simulink model "IARC_Nonlinear_Sensors"  (R2018a)
settings: Solver=ode1  StartTime=0.0  StopTime=20  FixedStep=T  RelTol=1e-3  EnableMultiTasking=on
undefined symbols (not defined in the file): A_1df, A_2df, alpha3, alpha_rp, alpha_x, alpha_z, an1, an1_v, an2, an3, bn1, bn1_v, bn2, bn3, dc_M_x, delta3, Epsilon3, F, g, Gamma1, Gamma2, Gamma3, Gamma4, gamma4_0, gamma_d_x, gamma_rp_0, gamma_x_0, gamma_z_0, Gammax, I, I_add, I_add_time, Jx, Jy, Jyaw, K, k1, k10, k11, k12, k2, k3, k4, k5, k6, k7, k8, k9, Ky, L, Light, LIMIT_CMD_PITCH, LIMIT_CMD_ROLL, LIMIT_CMD_xy, LIMIT_uCMD_HEIGHT, m, m_add, m_add_time, magnitude, MIL ... (+67)
libraries: simulink x131, simulink_extras x5, UAV_Control x4, aerolibwind2 x1
(part 4 of 6)

== system IARC_Nonlinear_Sensors/ARC Controller/Position Control/Z control/Estimate theta = K//m ==
  Phi_d : Inport
  error : Inport  Port=2
  f(f) : Inport  Port=3
  Phi : Inport  Port=4
  adappt : Inport  Port=5
  1 : Scope
  11 : Scope
  Constant4 : Constant  Value=6.7
  Constant6 : Constant  Value=theta3_Max(1,1)
  Constant7 : Constant  Value=theta3_Min(1,1)
  Demux1 : Demux  Outputs=2
  Demux2 : Demux  Outputs=2
  Gain1 : Gain  Gain=K
  "IARC, Physical Model Based Parameter Estimation (69)" : Subsystem  AncestorBlock=|  mask(Physical Model Based Parameter Estimation){mu1=mu1_z, mu2=mu2_z, alpha=alpha_z, nu=nu_z, gamma0=gamma_z_0, Rho_M=Rho_M_z, Rho_L=Rho_L_z, v=v_z, theta_0=theta3_0, theta_max=theta3_Max, theta_min=theta3_Min, Theta_dot_M=theta_dot_M_z, Tau=Tau_z, t0=t0, Norm_ON=on}
      | UAV_Control/IARC, Physical Model Based 
      | Parameter Estimation (69)
      mask prompts: mu1 "forgetting factor, mu1:"; mu2 "RLS parameter, mu2:"; alpha "forgetting factor, alpha:"; nu "normalizing factor, nu:"; gamma0 "Initial adaptation gain:"; Rho_M "Upper bound for the adaptation gain:"; Rho_L "Lower bound for the adaptation gain:"; v "Eigenvector of Gamma_max:"; Theta_dot_M "Theta dot max:"; Tau "Filter time constant:"; t0 "Initialization Delay:"; Norm_ON "Use Normalized formula"
      mask Help:
      | Filtered system dynamics:
      | H_f (s)  is any stable LTI filter transfer function
      | x_f=H_f [x]
      | φ_f=H_f [φ(x)]
      | u_f=H_f [u]
      | 
      | y_p=x ̇_f−u_f
      | y ̂_p=φ_f^T θ ̂
      | Prediction error:
      | ϵ=y_p−y ̂_p
      | 
      | recursive estimation algorithms, the generalized parameter estimation algorithm (PAA) with covariance limiting:
      | 
      | θ ̂  ̇(t)=Γ(t) φ_f (t)ϵ(t)
      | D_Γ=μ_1 (t)Γ(t)−μ_2 (t)Γ(t) φ_f (t) φ_f (t)^T Γ(t)
      | Γ ̇(t)=D_Γ, if λ_M (Γ(t))<ρ_M  or v_M^T D_Γ v_M<0 )
      |          0        else
      | 
      | μ_1  and μ_2  are two non-negative functions
      | ρ_M  is a preset upper bound for the covariance matrix Γ(t)
      | μ_1  represents the forgetting factor (μ_1=0 for not forgetting)
      | μ_2: 1 stands for the standard least squares type estimation algorithm
      |        0 stands for  the gradient type estimation algorithm
      |        range: 0≤μ_2<2
      | Initialization of the covariance matrix: Γ(0)<ρ_M I_p
      | 
      | IARC designs completely separate the parameter estimation law design from the underlying robust control law to give better parameter estimates than possible with DARC designs. In addition, explicit on-line signal excitation level monitoring can be employed to significantly improve the accuracy of  parameter estimates.
      | 
      | Normalized Method:
      | θ ̂  ̇(t)=(Γ(t) φ_f (t)ϵ(t))/(1+νφ_f^T Γφ_f )
      | D_Γ=αΓ(t)−(Γ(t) φ_f (t) φ_f (t)^T Γ(t))/(1+νφ_f^T Γφ_f )
      | Γ ̇(t)=D_Γ, if λ_M (Γ(t))<ρ_M  or v_M^T D_Γ v_M<0
      |           0       else
      mask Display:
      | port_label('input',1,'y','texmode','on')
      | port_label('input',2,'\phi','texmode','on')
      | port_label('input',3,'Adapt','texmode','on')
      | 
      | port_label('output',1,'\theta_{hat}','texmode','on')
  Integral Type Adaptation Law Discontinuous Projection : Subsystem  AncestorBlock=|  mask(IntegralTypeAdaptationLaw){theta=theta3(1,1), theta0=theta3_0(1,1), theta_max=theta3_Max(1,1), theta_min=theta3_Min(1,1), gamma=Gamma3(1,1), t0=3, Adaptation_ON=on}
      | UAV_Control/Integral Type
      | Adaptation Law
      | Discontinuous Projection
      mask prompts: theta "Actual value of theta:"; theta0 "Initial value of theta:"; theta_max "Maximum value of theta:"; theta_min "Minimum value of theta:"; gamma "Adaptation Rate:"; t0 "Initialization Delay:"; Adaptation_ON "Activate adaptation:"
      mask help: Applies an Integral-type adaptation law with discontinuous projection on the parameter theta.
      mask Help:
      | Applies an Integral-type adaptation law with discontinuous projection on the parameter theta.
      | 
      | theta_est_dot=Gamma*Phi*e
      | theta=proj( int(theta_estdot) )
      | 
      | theta_min < theta_est <  theta_max
      | 
      | Parameters:
      | 
      | Gamma: nxn diagonal matrix, adaptaion rate.
      | theta_min: nx1 vector, minimum value of the estimated vector.
      | theta_max: nx1 vector, maximum value of the estimated vector.
      | theta0: nx1 vector, initial value of the estimated vector.
      | theta: nx1 vector, actual value of the estimated vector.
      | Adaptation_On: controls the use of the adaptation law (1: active, 0: inactive)
      | 
      | Inputs:
      | Phi: regressor vector, theta0, nx1.
      | e: state error, scalar.
      | 
      | Outputs:
      | theta_est: estimated value of the parameters vector.
      mask Display:
      | port_label('input',1,'\phi','texmode','on')
      | port_label('input',2,'e','texmode','on')
      | port_label('output',1,'\theta_{hat}','texmode','on')
  Manual Switch : ManualSwitch  CurrentSetting=0
  Manual Switch1 : ManualSwitch
  Math Function1 : Math  Operator=reciprocal  SaturateOnIntegerOverflow=on
  Mux8 : Mux  Inputs=5
  To File : ToFile  Commented=on  Filename=IARC31.mat  MatrixName=IARC31  SaveFormat=Timeseries
  To Workspace2 : ToWorkspace  Commented=on  VariableName=theta_3  SaveFormat=Timeseries  SampleTime=-1
  m : Subsystem
  m (kg) : Scope
  theta1 : Outport
  theta2 : Outport  Port=2
  wires:
  Phi/1 -> "IARC, Physical Model Based Parameter Estimation (69)"/2(Phi)
  Constant6/1 -> Mux8/4
  Integral Type Adaptation Law Discontinuous Projection/1(theta_est) -> 11/1, Mux8/1, Manual Switch/1
  Demux2/1 -> Manual Switch/2, Mux8/2
  m/1(Out1) -> Mux8/3
  Math Function1/1 -> Gain1/1
  error/1 -> Integral Type Adaptation Law Discontinuous Projection/2(error)
  Manual Switch/1 -> 1/1, theta1/1, To Workspace2/1
  Constant7/1 -> Mux8/5
  Gain1/1 -> To File/1, m (kg)/1
  Mux8/1 -> Math Function1/1
  Phi_d/1 -> Integral Type Adaptation Law Discontinuous Projection/1(Phi)
  f(f)/1 -> "IARC, Physical Model Based Parameter Estimation (69)"/1(y)
  adappt/1 -> "IARC, Physical Model Based Parameter Estimation (69)"/3(Adapt1)
  Manual Switch1/1 -> theta2/1
  "IARC, Physical Model Based Parameter Estimation (69)"/1(Theta_hat) -> Demux2/1
  Demux1/2 -> Manual Switch1/1
  Demux2/2 -> Manual Switch1/2

== system IARC_Nonlinear_Sensors/ARC Controller/Position Control/Z control/Phi ==
  "  " : Gain  Gain=1/K
  Constant : Constant
  Mux1 : Mux  Inputs=2
  Mux2 : Mux  Inputs=2
  Product1 : Product
  cos : Trigonometry  Operator=cos
  cos(phi).cos(theta) : Fcn  Expr=u(1)*u(2)
  rotor TF : TransferFcn  Numerator=1  Denominator=[Tm 1]
  Out1 : Outport
  wires:
  Mux2/1 -> cos/1
  [phi] -> Mux2/1
  cos(phi).cos(theta)/1 -> Product1/1
  [theta] -> Mux2/2
  rotor TF/1 -> Product1/2
  Mux1/1 -> Out1/1
  Product1/1 -> Mux1/1
  Constant/1 -> Mux1/2
  [Fz_des] -> "  "/1
  cos/1 -> cos(phi).cos(theta)/1
  "  "/1 -> rotor TF/1

== system IARC_Nonlinear_Sensors/ARC Controller/Position Control/Z control/Phi1 ==
  "  " : Gain  Gain=1/K
  Fcn33 : Fcn  Expr=u(4)*u(5)
  Mux : Mux  Inputs=2
  Mux2 : Mux  Inputs=3
  Product1 : Product
  rotor2 : TransferFcn  Numerator=1  Denominator=[Tm 1]
  sincos : Trigonometry  Operator=sincos
  Out1 : Outport
  wires:
  Product1/1 -> Out1/1
  rotor2/1 -> Product1/2
  [theta] -> Mux2/2
  Fcn33/1 -> Product1/1
  sincos/1 -> Mux/1
  sincos/2 -> Mux/2
  [psi] -> Mux2/3
  Mux/1 -> Fcn33/1
  [phi] -> Mux2/1
  Mux2/1 -> sincos/1
  [Fz_des] -> "  "/1
  "  "/1 -> rotor2/1

== system IARC_Nonlinear_Sensors/ARC Controller/Position Control/Z control/Phi3 ==
  "  " : Gain  Gain=1/K
  Constant : Constant
  Mux1 : Mux  Inputs=2
  Mux2 : Mux  Inputs=2
  Product1 : Product
  cos : Trigonometry  Operator=cos
  cos(phi).cos(theta) : Fcn  Expr=u(1)*u(2)
  rotor TF : TransferFcn  Numerator=1  Denominator=[Tm 1]
  Out1 : Outport
  wires:
  cos/1 -> cos(phi).cos(theta)/1
  [Fz_des] -> "  "/1
  Constant/1 -> Mux1/2
  Product1/1 -> Mux1/1
  Mux1/1 -> Out1/1
  rotor TF/1 -> Product1/2
  [theta] -> Mux2/2
  cos(phi).cos(theta)/1 -> Product1/1
  [phi] -> Mux2/1
  Mux2/1 -> cos/1
  "  "/1 -> rotor TF/1

== system IARC_Nonlinear_Sensors/ARC Controller/Position Control/Z control/e10 ==
  Add : Sum
  Discrete Derivative2 : simulink/Discrete/Discrete Derivative  gainval=1.0  ICPrevScaledInput=0.0  OutMin=[]  OutMax=[]  OutDataType=fixdt(1, 16)  OutScaling=2^-10  DoSatur=off
  Sum1 : Sum  Inputs=-+|
  Sum3 : Sum  Inputs=|+-
  k9 : Gain  Gain=k9
  e10 : Outport
  wires:
  k9/1 -> Add/1
  Discrete Derivative2/1 -> Sum1/1
  [z_dot] -> Sum1/2
  Add/1 -> e10/1
  Sum3/1 -> k9/1  "ex"
  Sum1/1 -> Add/2  "ev"
  [z] -> Sum3/1
  [z_des] -> Discrete Derivative2/1, Sum3/2

== system IARC_Nonlinear_Sensors/ARC Controller/Position Control/Z control/f(x) ==
  Add : Sum
  Constant : Constant  Value=g
  Discrete Derivative1 : simulink/Discrete/Discrete Derivative  gainval=1.0  ICPrevScaledInput=0.0  OutMin=[]  OutMax=[]  OutDataType=fixdt(1, 16)  OutScaling=2^-10  DoSatur=off
  Out1 : Outport
  wires:
  Add/1 -> Out1/1
  [z_dot] -> Discrete Derivative1/1
  Discrete Derivative1/1 -> Add/1
  Constant/1 -> Add/2

== system IARC_Nonlinear_Sensors/Sensors and Filters/Data processing/Estimate Attitude/2nd Order Filter3 ==
  u : Inport
  "  1" : Constant  Value=OMEGA_FILTER_OUTER
  "  2" : Constant  Value=2
  "  zea" : Constant
  Integrator : Integrator
  Integrator1 : Integrator
  Product : Product
  Product1 : Product
  Product2 : Product  Inputs=3
  Sum : Sum  Inputs=|+-
  Sum1 : Sum  Inputs=|+-
  y : Outport
  yd : Outport  Port=2
  wires:
  Product2/1 -> Sum1/2
  "  zea"/1 -> Product2/3
  "  2"/1 -> Product2/2
  Product1/1 -> Integrator1/1, yd/1
  Integrator1/1 -> y/1, Sum/2
  u/1 -> Sum/1
  Sum1/1 -> Product/2
  "  1"/1 -> Product/1, Product1/1
  Product/1 -> Integrator/1
  Integrator/1 -> Product1/2, Product2/1
  Sum/1 -> Sum1/1

== system IARC_Nonlinear_Sensors/Sensors and Filters/Data processing/Estimate Attitude/Calculate Roll and Pitch (From Acceleration Data) ==
  accel (m/s^2) [3] : Inport
  Gain{1..2,6..7} (4 alike) : Gain  Commented=on  Gain=180/pi
  Gain3 : Gain
  calc_roll_pitch : MATLAB Function  TreatAsAtomicUnit=on
  calc_roll_pitch_asin : MATLAB Function  Commented=on  TreatAsAtomicUnit=on
  pitch_acc : Scope  Commented=on
  pitch_acc_asin : Scope  Commented=on
  roll_acc : Scope  Commented=on
  roll_acc_asin : Scope  Commented=on
  roll_acc (rad) : Outport
  pitch_acc (rad) : Outport  Port=2
  wires:
  accel (m/s^2) [3]/1 -> calc_roll_pitch_asin/1(acc_body), calc_roll_pitch/1(acc_body)
  calc_roll_pitch/1(roll_acc) -> roll_acc (rad)/1, Gain2/1
  calc_roll_pitch/2(pitch_acc) -> Gain3/1, Gain1/1
  Gain2/1 -> roll_acc/1
  Gain1/1 -> pitch_acc/1
  calc_roll_pitch_asin/1(roll_acc) -> Gain6/1
  Gain6/1 -> roll_acc_asin/1
  calc_roll_pitch_asin/2(pitch_acc) -> Gain7/1
  Gain7/1 -> pitch_acc_asin/1
  Gain3/1 -> pitch_acc (rad)/1

== system IARC_Nonlinear_Sensors/Sensors and Filters/Data processing/Estimate Attitude/Notch Filter1 ==
  u : Inport
  Discrete Transfer Fcn : DiscreteTransferFcn  Numerator=an1  Denominator=bn1  SampleTime=1/500
  Discrete Transfer Fcn1 : DiscreteTransferFcn  Numerator=an2  Denominator=bn2  SampleTime=1/500
  Discrete Transfer Fcn2 : DiscreteTransferFcn  Numerator=an3  Denominator=bn3  SampleTime=1/500
  First-Order Hold : simulink/Discrete/First-Order Hold  DisableCoverage=on  Ts=1/500
      settings: SourceProductName=Simulink  SourceProductBaseCode=SL
  Mux : Mux  Commented=on
  Mux1 : Mux  Commented=on  Inputs=2
  Scope : Scope  Commented=on
  Scope1 : Scope  Commented=on
  Transfer Fcn : TransferFcn  Numerator=[60]  Denominator=[1 60]
  y : Outport
  q : Outport  Port=2
  wires:
  u/1 -> Mux1/1, Transfer Fcn/1
  Transfer Fcn/1 -> Mux1/2, First-Order Hold/1, y/1
  Discrete Transfer Fcn1/1 -> Mux/3, Discrete Transfer Fcn2/1
  First-Order Hold/1 -> Discrete Transfer Fcn/1, Mux/1
  Mux/1 -> Scope/1
  Discrete Transfer Fcn/1 -> Mux/2, Discrete Transfer Fcn1/1
  Mux1/1 -> Scope1/1
  Discrete Transfer Fcn2/1 -> q/1, Mux/4

== system IARC_Nonlinear_Sensors/Sensors and Filters/Data processing/Estimate Attitude/Notch Filter2 ==
  u : Inport
  Discrete Transfer Fcn : DiscreteTransferFcn  Numerator=an1  Denominator=bn1  SampleTime=1/500
  Discrete Transfer Fcn1 : DiscreteTransferFcn  Numerator=an2  Denominator=bn2  SampleTime=1/500
  Discrete Transfer Fcn2 : DiscreteTransferFcn  Numerator=an3  Denominator=bn3  SampleTime=1/500
  First-Order Hold : simulink/Discrete/First-Order Hold  DisableCoverage=on  Ts=1/500
      settings: SourceProductName=Simulink  SourceProductBaseCode=SL
  Mux : Mux  Commented=on
  Mux1 : Mux  Commented=on  Inputs=2
  Scope : Scope  Commented=on
  Scope1 : Scope  Commented=on
  To File : ToFile  Commented=on  Filename=P_gyro_Noisy.mat  MatrixName=P_gyro_Noisy  SaveFormat=Timeseries
  Transfer Fcn : TransferFcn  Numerator=[60]  Denominator=[1 60]
  y : Outport
  p : Outport  Port=2
  wires:
  Mux1/1 -> Scope1/1
  Discrete Transfer Fcn/1 -> Discrete Transfer Fcn1/1, Mux/2
  Discrete Transfer Fcn2/1 -> p/1, Mux/4
  Mux/1 -> Scope/1
  First-Order Hold/1 -> Mux/1, Discrete Transfer Fcn/1
  Discrete Transfer Fcn1/1 -> Discrete Transfer Fcn2/1, Mux/3
  Transfer Fcn/1 -> y/1, First-Order Hold/1, Mux1/2
  u/1 -> To File/1, Transfer Fcn/1, Mux1/1

== system IARC_Nonlinear_Sensors/Sensors and Filters/Data processing/Estimate Attitude/Notch Filter3 ==
  u : Inport
  Discrete Transfer Fcn : DiscreteTransferFcn  Numerator=an1  Denominator=bn1  SampleTime=1/500
  Discrete Transfer Fcn1 : DiscreteTransferFcn  Numerator=an2  Denominator=bn2  SampleTime=1/500
  Discrete Transfer Fcn2 : DiscreteTransferFcn  Numerator=an3  Denominator=bn3  SampleTime=1/500
  First-Order Hold : simulink/Discrete/First-Order Hold  DisableCoverage=on  Ts=1/500
      settings: SourceProductName=Simulink  SourceProductBaseCode=SL
  Mux : Mux  Commented=on
  Mux1 : Mux  Commented=on  Inputs=2
  Scope : Scope  Commented=on
  Scope1 : Scope  Commented=on
  Transfer Fcn : TransferFcn  Numerator=[60]  Denominator=[1 60]
  y : Outport
  r : Outport  Port=2
  wires:
  u/1 -> Mux1/1, Transfer Fcn/1
  Transfer Fcn/1 -> Mux1/2, First-Order Hold/1, y/1
  Discrete Transfer Fcn1/1 -> Mux/3, Discrete Transfer Fcn2/1
  First-Order Hold/1 -> Discrete Transfer Fcn/1, Mux/1
  Mux/1 -> Scope/1
  Discrete Transfer Fcn2/1 -> r/1, Mux/4
  Discrete Transfer Fcn/1 -> Mux/2, Discrete Transfer Fcn1/1
  Mux1/1 -> Scope1/1

== system IARC_Nonlinear_Sensors/Sensors and Filters/Data processing/Estimate Position/2nd Order Filter ==
  u : Inport
  "  2" : Constant  Value=2
  "  wn" : Constant  Value=OMEGA_FILTER_OUTER
  "  zea" : Constant
  Integrator : Integrator
  Integrator1 : Integrator
  Product : Product
  Product1 : Product
  Product2 : Product  Inputs=3
  Sum : Sum  Inputs=|+-
  Sum1 : Sum  Inputs=|+-
  y : Outport
  yd : Outport  Port=2
  wires:
  Sum/1 -> Sum1/1
  Integrator/1 -> Product2/1, Product1/2
  Product/1 -> Integrator/1
  "  wn"/1 -> Product1/1, Product/1
  Sum1/1 -> Product/2
  u/1 -> Sum/1
  Integrator1/1 -> Sum/2, y/1
  Product1/1 -> yd/1, Integrator1/1
  "  2"/1 -> Product2/2
  "  zea"/1 -> Product2/3
  Product2/1 -> Sum1/2

== system IARC_Nonlinear_Sensors/Sensors and Filters/Data processing/Estimate Position/2nd Order Filter1 ==
  u : Inport
  "  2" : Constant  Value=2
  "  wn" : Constant  Value=OMEGA_FILTER_OUTER
  "  zea" : Constant
  Integrator : Integrator
  Integrator1 : Integrator
  Product : Product
  Product1 : Product
  Product2 : Product  Inputs=3
  Sum : Sum  Inputs=|+-
  Sum1 : Sum  Inputs=|+-
  y : Outport
  yd : Outport  Port=2
  wires:
  Product2/1 -> Sum1/2
  "  zea"/1 -> Product2/3
  "  2"/1 -> Product2/2
  Product1/1 -> Integrator1/1, yd/1
  Integrator1/1 -> y/1, Sum/2
  u/1 -> Sum/1
  Sum1/1 -> Product/2
  "  wn"/1 -> Product/1, Product1/1
  Product/1 -> Integrator/1
  Integrator/1 -> Product1/2, Product2/1
  Sum/1 -> Sum1/1

== system IARC_Nonlinear_Sensors/Sensors and Filters/Data processing/Estimate Position/2nd Order Filter2 ==
  u : Inport
  "  2" : Constant  Value=2
  "  wn" : Constant  Value=OMEGA_FILTER_OUTER
  "  zea" : Constant
  Integrator : Integrator
  Integrator1 : Integrator
  Product : Product
  Product1 : Product
  Product2 : Product  Inputs=3
  Sum : Sum  Inputs=|+-
  Sum1 : Sum  Inputs=|+-
  y : Outport
  yd : Outport  Port=2
  wires:
  Sum/1 -> Sum1/1
  Integrator/1 -> Product2/1, Product1/2
  Product/1 -> Integrator/1
  "  wn"/1 -> Product1/1, Product/1
  Sum1/1 -> Product/2
  u/1 -> Sum/1
  Integrator1/1 -> Sum/2, y/1
  Product1/1 -> yd/1, Integrator1/1
  "  2"/1 -> Product2/2
  "  zea"/1 -> Product2/3
  Product2/1 -> Sum1/2

== system IARC_Nonlinear_Sensors/Sensors and Filters/Data processing/Estimate Position/2nd Order Filter4 ==
  u : Inport
  "  1" : Constant  Value=OMEGA_FILTER_OUTER
  "  2" : Constant  Value=2
  "  zea" : Constant
  Integrator : Integrator
  Integrator1 : Integrator
  Product : Product
  Product1 : Product
  Product2 : Product  Inputs=3
  Sum : Sum  Inputs=|+-
  Sum1 : Sum  Inputs=|+-
  y : Outport
  yd : Outport  Port=2
  wires:
  Product2/1 -> Sum1/2
  "  zea"/1 -> Product2/3
  "  2"/1 -> Product2/2
  Product1/1 -> Integrator1/1, yd/1
  Integrator1/1 -> y/1, Sum/2
  u/1 -> Sum/1
  Sum1/1 -> Product/2
  "  1"/1 -> Product/1, Product1/1
  Product/1 -> Integrator/1
  Integrator/1 -> Product1/2, Product2/1
  Sum/1 -> Sum1/1

== system IARC_Nonlinear_Sensors/Sensors and Filters/Data processing/Estimate Position/2nd Order Filter5 ==
  u : Inport
  "  2" : Constant  Value=2
  "  wn" : Constant  Value=OMEGA_FILTER_OUTER
  "  zea" : Constant
  Integrator : Integrator
  Integrator1 : Integrator
  Product : Product
  Product1 : Product
  Product2 : Product  Inputs=3
  Sum : Sum  Inputs=|+-
  Sum1 : Sum  Inputs=|+-
  y : Outport
  yd : Outport  Port=2
  wires:
  Product2/1 -> Sum1/2
  "  zea"/1 -> Product2/3
  "  2"/1 -> Product2/2
  Product1/1 -> Integrator1/1, yd/1
  Integrator1/1 -> y/1, Sum/2
  u/1 -> Sum/1
  Sum1/1 -> Product/2
  "  wn"/1 -> Product/1, Product1/1
  Product/1 -> Integrator/1
  Integrator/1 -> Product1/2, Product2/1
  Sum/1 -> Sum1/1

== system IARC_Nonlinear_Sensors/Sensors and Filters/Data processing/Estimate Position/Notch Filter1 ==
  u : Inport
  Discrete Transfer Fcn : DiscreteTransferFcn  Numerator=an1_v  Denominator=bn1_v  SampleTime=1/500
  First-Order Hold : simulink/Discrete/First-Order Hold  DisableCoverage=on  Ts=1/500
      settings: SourceProductName=Simulink  SourceProductBaseCode=SL
  Mux : Mux  Commented=on  Inputs=3
  Scope : Scope  Commented=on
  Transfer Fcn : TransferFcn  Numerator=[60]  Denominator=[1 60]
  y : Outport
  wires:
  u/1 -> Transfer Fcn/1, Mux/1
  First-Order Hold/1 -> Discrete Transfer Fcn/1, Mux/2
  Mux/1 -> Scope/1
  Discrete Transfer Fcn/1 -> y/1, Mux/3
  Transfer Fcn/1 -> First-Order Hold/1

== system IARC_Nonlinear_Sensors/Sensors and Filters/Data processing/Estimate Position/Notch Filter2 ==
  u : Inport
  Discrete Transfer Fcn : DiscreteTransferFcn  Numerator=an1_v  Denominator=bn1_v  SampleTime=1/500
  First-Order Hold : simulink/Discrete/First-Order Hold  DisableCoverage=on  Ts=1/500
      settings: SourceProductName=Simulink  SourceProductBaseCode=SL
  Mux : Mux  Commented=on  Inputs=3
  Scope : Scope  Commented=on
  Transfer Fcn : TransferFcn  Numerator=[60]  Denominator=[1 60]
  y : Outport
  wires:
  Discrete Transfer Fcn/1 -> y/1, Mux/3
  Mux/1 -> Scope/1
  First-Order Hold/1 -> Mux/2, Discrete Transfer Fcn/1
  u/1 -> Mux/1, Transfer Fcn/1
  Transfer Fcn/1 -> First-Order Hold/1

== system IARC_Nonlinear_Sensors/Sensors and Filters/Data processing/Estimate Position/Signal Conditioning - Sonar ==
  note: Correct for Roll and Pitch
  note: "Smooth" out the Sonar data
  note: Resample the 10Hz Sonar Data
  sonar (m) : Inport
  roll (rad) : Inport  Port=2
  pitch (rad) : Inport  Port=3
  FOH1 : Subsystem  mask{Ts=0.1}
      mask prompts: Ts "Sample Time"
  "Height Estimate Bias (Estimate Reference at Centre of QBall 2) " : Bias
  Product : Product  Inputs=3  RndMeth=Zero
  Rate Transition : RateTransition
  Sampler : Subsystem  mask{Ts=0.1}
      mask prompts: Ts "Sample Time"
  Trigonometric Function : Trigonometry  Operator=cos
  Trigonometric Function2 : Trigonometry  Operator=cos
  calib sonar (m) : Outport
  wires:
  Sampler/1(Out1) -> Rate Transition/1
  Rate Transition/1 -> FOH1/1(Input)
  sonar (m)/1 -> Sampler/1(In1)
  FOH1/1(Output) -> Product/1
  Trigonometric Function2/1 -> Product/2
  roll (rad)/1 -> Trigonometric Function2/1
  pitch (rad)/1 -> Trigonometric Function/1
  Trigonometric Function/1 -> Product/3
  Product/1 -> "Height Estimate Bias (Estimate Reference at Centre of QBall 2) "/1
  "Height Estimate Bias (Estimate Reference at Centre of QBall 2) "/1 -> calib sonar (m)/1

== system IARC_Nonlinear_Sensors/ARC Controller/Attitutde Control/Subsystem/f/d(T)//d(phi) ==
  R1,R2,R3 : Inport  PortDimensions=3
  Fcn{1,11..13,22,32} (6 alike) : Fcn  Expr=0
  Fcn2 : Fcn  Expr=u(4)
  Fcn3 : Fcn  Expr=-u(1)*u(5)
  Fcn31 : Fcn  Expr=u(1)*u(2)
  Mux : Mux  Inputs=2
  Subsystem : Subsystem
  sincos : Trigonometry  Operator=sincos
  T : Outport  PortDimensions=[3,3]
  wires:
  Fcn3/1 -> Subsystem/9(In9)
  Fcn2/1 -> Subsystem/8(In8)
  Fcn1/1 -> Subsystem/6(In6)
  Fcn22/1 -> Subsystem/5(In5)
  Fcn31/1 -> Subsystem/7(In7)
  Fcn32/1 -> Subsystem/4(In4)
  Fcn13/1 -> Subsystem/3(In3)
  Fcn12/1 -> Subsystem/2(In2)
  Fcn11/1 -> Subsystem/1(In1)
  Mux/1 -> Fcn1/1, Fcn31/1, Fcn3/1, Fcn2/1, Fcn32/1, Fcn12/1, Fcn11/1, Fcn13/1, Fcn22/1
  sincos/2 -> Mux/2
  sincos/1 -> Mux/1
  Subsystem/1(Out1) -> T/1
  R1,R2,R3/1 -> sincos/1

== system IARC_Nonlinear_Sensors/ARC Controller/Attitutde Control/Subsystem/f/d(T)//d(theta) ==
  R1,R2,R3 : Inport  PortDimensions=3
  Fcn{1..2,12,22,32} (5 alike) : Fcn  Expr=0
  Fcn11 : Fcn  Expr=-u(2)
  Fcn13 : Fcn  Expr=u(5)
  Fcn3 : Fcn  Expr=-u(4)*u(2)
  Fcn31 : Fcn  Expr=-u(4)*u(5)
  Mux : Mux  Inputs=2
  Subsystem : Subsystem
  sincos : Trigonometry  Operator=sincos
  T : Outport  PortDimensions=[3,3]
  wires:
  R1,R2,R3/1 -> sincos/1
  Subsystem/1(Out1) -> T/1
  sincos/1 -> Mux/1
  sincos/2 -> Mux/2
  Mux/1 -> Fcn22/1, Fcn13/1, Fcn11/1, Fcn12/1, Fcn32/1, Fcn2/1, Fcn3/1, Fcn31/1, Fcn1/1
  Fcn11/1 -> Subsystem/1(In1)
  Fcn12/1 -> Subsystem/2(In2)
  Fcn13/1 -> Subsystem/3(In3)
  Fcn32/1 -> Subsystem/4(In4)
  Fcn31/1 -> Subsystem/7(In7)
  Fcn22/1 -> Subsystem/5(In5)
  Fcn1/1 -> Subsystem/6(In6)
  Fcn2/1 -> Subsystem/8(In8)
  Fcn3/1 -> Subsystem/9(In9)

== system IARC_Nonlinear_Sensors/ARC Controller/Attitutde Control/Yaw control/Phi3/alpha 42 dot ==
  Add : Sum  Inputs=-+
  Discrete Derivative1 : simulink/Discrete/Discrete Derivative  gainval=1.0  ICPrevScaledInput=0.0  OutMin=[]  OutMax=[]  OutDataType=fixdt(1, 16)  OutScaling=2^-10  DoSatur=off
  Discrete Derivative2 : simulink/Discrete/Discrete Derivative  gainval=1.0  ICPrevScaledInput=0.0  OutMin=[]  OutMax=[]  OutDataType=fixdt(1, 16)  OutScaling=2^-10  DoSatur=off
  Sum3 : Sum  Inputs=|+-
  Transfer Fcn3 : TransferFcn  Denominator=A_2df
  k11 : Gain  Gain=k11
  alpha_42_dot : Outport
  wires:
  [psi_des] -> Sum3/2, Discrete Derivative2/1
  [psi] -> Sum3/1
  Sum3/1 -> k11/1  "ex"
  Add/1 -> alpha_42_dot/1
  Discrete Derivative2/1 -> Discrete Derivative1/1
  k11/1 -> Add/1
  Transfer Fcn3/1 -> Add/2
  Discrete Derivative1/1 -> Transfer Fcn3/1

== system IARC_Nonlinear_Sensors/ARC Controller/Attitutde Control/Yaw control/Subsystem/  ==
  1 : Scope  Commented=on
  Constant4 : Constant  Value=Jyaw
  Divide : Product  Inputs=*/
  J_add : Step  Time=I_add_time  After=I_add(3,3)  SampleTime=0
  Selector : Selector  InputPortWidth=3  IndexOptions=Index vector (dialog)  Indices=3  OutputSizes=1
  Sum : Sum  Inputs=|++
  Sum1 : Sum  Inputs=++|
  T_add : Step  Time=T_add_time  After=T_add(1,3)  SampleTime=0
  Out1 : Outport
  wires:
  T_add/1 -> Sum1/2
  [Md] -> Selector/1
  Divide/1 -> 1/1, Out1/1
  Sum/1 -> Divide/2
  Constant4/1 -> Sum/1
  J_add/1 -> Sum/2
  Sum1/1 -> Divide/1
  Selector/1 -> Sum1/1

== system IARC_Nonlinear_Sensors/ARC Controller/Attitutde Control/Yaw control/Subsystem/IARC, Physical Model Based Parameter Estimation (69)_Yaw ==
  f(x) : Inport
  Phi : Inport  Port=2
  Adapt : Inport  Port=3
  Adapt1 : InportShadow  Port=3
  Constant2 : Constant  Value=Norm_ON
  Discontinuous_Proj_(49) : Subsystem
  Display : Display  Commented=on
  Divide : Product  Inputs=*/
  Epsilon : Subsystem
  Filter : Subsystem
  Gamma : Subsystem
  Switch1 : Switch  Threshold=0.5
  Theta_hat_dot : Product  Inputs=3  Multiplication=Matrix(*)
  den : Scope  Commented=on
  "epsilon  " : Scope  Commented=on
  gamma : Scope  Commented=on
  theta dot : Scope  Commented=on
  theta hat : Scope  Commented=on
  Theta_hat : Outport
  wires:
  Epsilon/1(Epsilon) -> Theta_hat_dot/3, "epsilon  "/1  "predicted output error"
  Discontinuous_Proj_(49)/1(Theta) -> theta hat/1, Theta_hat/1, Epsilon/3(Theta_hat)
  Filter/1(f(x)_f) -> Epsilon/1(f(x)_f_dot)
  Phi/1 -> Filter/2("Phi ")
  f(x)/1 -> Filter/1(f(x))
  Theta_hat_dot/1 -> Discontinuous_Proj_(49)/1(Theta_dot), theta dot/1
  Constant2/1 -> Switch1/2
  Gamma/1(" gamma") -> Display/1, gamma/1, Switch1/3, Divide/1
  Switch1/1 -> Theta_hat_dot/1
  Divide/1 -> Switch1/1
  Gamma/2(" 1+nu.Phi.G.Phi") -> den/1, Divide/2
  Filter/2(Phi_f) -> Epsilon/2(Phi_f), Gamma/1(Phi_f), Theta_hat_dot/2
  Adapt/1 -> Gamma/2(Adapt)
  Adapt1/1 -> Discontinuous_Proj_(49)/2(Adapt)

== system IARC_Nonlinear_Sensors/ARC Controller/Attitutde Control/Yaw control/Subsystem/Integral Type Adaptation Law Discontinuous Projection1 ==
  Phi : Inport
  error : Inport  Port=2
  Constant : Constant  Value=gamma
  Constant2 : Constant  Value=Adaptation_ON
  Discontinuous Projection : Integrator  InitialCondition=theta0  LimitOutput=on  UpperSaturationLimit=theta_max  LowerSaturationLimit=theta_min
  InitializationDelay : UAV_Control/InitializationDelay  t0=t0
      settings: SourceProductName=UAV_Control
  Product1 : Product  Inputs=3  Multiplication=Matrix(*)
  Switch1 : Switch  Criteria=u2 ~= 0
  real : Constant  Value=theta
  theta_est : Outport
  wires:
  Constant/1 -> Product1/1
  error/1 -> Product1/3
  real/1 -> Switch1/3
  Constant2/1 -> Switch1/2
  InitializationDelay/1 -> Discontinuous Projection/1
  Product1/1 -> InitializationDelay/1
  Phi/1 -> Product1/2
  Discontinuous Projection/1 -> Switch1/1
  Switch1/1 -> theta_est/1

== system IARC_Nonlinear_Sensors/ARC Controller/Attitutde Control/Yaw control/Subsystem/J ==
  Constant4 : Constant  Value=Jyaw
  Gain : Gain  Gain=Ky
  Math Function : Math  Operator=reciprocal  SaturateOnIntegerOverflow=on
  Step : Step  Time=I_add_time  After=I_add(3,3)  SampleTime=0
  Sum : Sum  Inputs=|++
  Out1 : Outport
  wires:
  Constant4/1 -> Sum/1
  Step/1 -> Sum/2
  Math Function/1 -> Gain/1
  Gain/1 -> Out1/1
  Sum/1 -> Math Function/1

== system IARC_Nonlinear_Sensors/ARC Controller/Attitutde Control/Yaw control/Subsystem/Subsystem1 ==
  u : Inport
  6 : Scope
  Constant4 : Constant  Value=Jy
  Divide : Product  Inputs=**
  J_add : Step  Time=I_add_time  After=I_add(1,1)  SampleTime=0
  Sum : Sum  Inputs=|++
  y : Outport
  wires:
  u/1 -> Divide/1
  J_add/1 -> Sum/2
  Divide/1 -> y/1
  Sum/1 -> Divide/2, 6/1
  Constant4/1 -> Sum/1

== system IARC_Nonlinear_Sensors/ARC Controller/Attitutde Control/Yaw control/f(x)/T1 .. ==
  "  " : Trigonometry  Operator=cos
  "    " : Trigonometry
  Constant : Constant  Value=Jx
  Gain1 : Gain  Gain=-1
  Product1 : Product  Inputs=*/*/
  Out1 : Outport
  wires:
  Product1/1 -> Gain1/1
  Gain1/1 -> Out1/1
  [T1] -> Product1/3
  Constant/1 -> Product1/4
  [phi] -> "  "/1
  [theta] -> "    "/1
  "  "/1 -> Product1/2
  "    "/1 -> Product1/1

== system IARC_Nonlinear_Sensors/ARC Controller/Attitutde Control/Yaw control/f(x)/f ==
  " " : Trigonometry  Operator=sincos
  "  " : Trigonometry
  "      " : Trigonometry  Operator=cos
  Add : Sum  Inputs=++-
  Add1 : Sum  Inputs=+-
  Constant1 : Constant  Value=(Jy-Jyaw)/Jx
  Discrete Derivative1 : simulink/Discrete/Discrete Derivative  gainval=1.0  ICPrevScaledInput=0.0  OutMin=[]  OutMax=[]  OutDataType=fixdt(1, 16)  OutScaling=2^-10  DoSatur=off
  Discrete Derivative2 : simulink/Discrete/Discrete Derivative  gainval=1.0  ICPrevScaledInput=0.0  OutMin=[]  OutMax=[]  OutDataType=fixdt(1, 16)  OutScaling=2^-10  DoSatur=off
  Discrete Derivative3 : simulink/Discrete/Discrete Derivative  gainval=1.0  ICPrevScaledInput=0.0  OutMin=[]  OutMax=[]  OutDataType=fixdt(1, 16)  OutScaling=2^-10  DoSatur=off
  Ground : Ground
  Product1 : Product
  Product2 : Product  Inputs=**/
  Product4 : Product  Inputs=***/
  Selector1 : Selector  InputPortWidth=3  IndexOptions=Index vector (dialog)  Indices=[2 3]  OutputSizes=1
  q.r : Product  Inputs=*
  Out1 : Outport
  wires:
  [phi] -> "      "/1
  "      "/1 -> Product4/4
  Product4/1 -> Add/2
  q.r/1 -> Product4/2
  Selector1/1 -> q.r/1
  [pqr_est] -> Selector1/1
  Constant1/1 -> Product4/1
  Discrete Derivative1/1 -> Product2/1
  " "/2 -> Product2/3
  Add1/1 -> Product2/2
  Product1/1 -> Add1/2
  " "/1 -> Product1/2
  Discrete Derivative2/1 -> Product1/1
  Discrete Derivative3/1 -> Add1/1
  [phi] -> " "/1, Discrete Derivative1/1
  Add/1 -> Out1/1
  Product2/1 -> Add/1
  [theta] -> "  "/1
  "  "/1 -> Product4/3
  [psi] -> Discrete Derivative2/1
  [theta] -> Discrete Derivative3/1
  Ground/1 -> Add/3

== system IARC_Nonlinear_Sensors/ARC Controller/Attitutde Control/Yaw control/phi/Notch Filter2 ==
  u : Inport
  Discrete Transfer Fcn : DiscreteTransferFcn  Numerator=an1  Denominator=bn1  SampleTime=1/500
  Discrete Transfer Fcn1 : DiscreteTransferFcn  Numerator=an2  Denominator=bn2  SampleTime=1/500
  Discrete Transfer Fcn2 : DiscreteTransferFcn  Numerator=an3  Denominator=bn3  SampleTime=1/500
  First-Order Hold : simulink/Discrete/First-Order Hold  DisableCoverage=on  Ts=1/500
      settings: SourceProductName=Simulink  SourceProductBaseCode=SL
  Mux : Mux
  Mux1 : Mux  Inputs=2
  Scope : Scope
  Scope1 : Scope
  Transfer Fcn : TransferFcn  Numerator=[60]  Denominator=[1 60]
  p : Outport
  wires:
  Mux1/1 -> Scope1/1
  Discrete Transfer Fcn/1 -> Discrete Transfer Fcn1/1, Mux/2
  Discrete Transfer Fcn2/1 -> p/1, Mux/4
  Mux/1 -> Scope/1
  First-Order Hold/1 -> Mux/1, Discrete Transfer Fcn/1
  Discrete Transfer Fcn1/1 -> Discrete Transfer Fcn2/1, Mux/3
  Transfer Fcn/1 -> First-Order Hold/1, Mux1/2
  u/1 -> Transfer Fcn/1, Mux1/1

== system IARC_Nonlinear_Sensors/ARC Controller/Attitutde Control/pitch control/Adaptation Law_X/  ==
  1 : Scope
  Constant4 : Constant  Value=Jy
  Divide : Product  Inputs=*/
  J_add : Step  Time=I_add_time  After=I_add(1,1)  SampleTime=0
  Selector : Selector  InputPortWidth=3  IndexOptions=Index vector (dialog)  Indices=2  OutputSizes=1
  Sum : Sum  Inputs=|++
  Sum1 : Sum  Inputs=++|
  T_add : Step  Time=T_add_time  After=T_add(1,2)  SampleTime=0
  Out1 : Outport
  wires:
  T_add/1 -> Sum1/2
  [Md] -> Selector/1
  Divide/1 -> 1/1, Out1/1
  Sum/1 -> Divide/2
  Constant4/1 -> Sum/1
  J_add/1 -> Sum/2
  Sum1/1 -> Divide/1
  Selector/1 -> Sum1/1

== system IARC_Nonlinear_Sensors/ARC Controller/Attitutde Control/pitch control/Adaptation Law_X/IARC, Physical Model Based Parameter Estimation (69)_pitch (theta) ==
  f(x) : Inport
  Phi : Inport  Port=2
  Adapt : Inport  Port=3
  Adapt1 : InportShadow  Port=3
  Constant2 : Constant  Value=Norm_ON
  Discontinuous_Proj_(49) : Subsystem
  Display : Display  Commented=on
  Divide : Product  Inputs=*/
  Epsilon : Subsystem
  Filter : Subsystem
  Gamma : Subsystem
  Switch1 : Switch  Threshold=0.5
  Theta_hat_dot : Product  Inputs=3  Multiplication=Matrix(*)
  Uf : Scope  Commented=on
  "epsilon  " : Scope  Commented=on
  gamma : Scope  Commented=on
  theta dot : Scope  Commented=on
  theta hat : Scope  Commented=on
  Theta_hat : Outport
  wires:
  Epsilon/1(Epsilon) -> Theta_hat_dot/3, "epsilon  "/1  "predicted output error"
  Discontinuous_Proj_(49)/1(Theta) -> theta hat/1, Theta_hat/1, Epsilon/3(Theta_hat)
  Filter/1(f(x)_f) -> Epsilon/1(f(x)_f_dot)
  Phi/1 -> Filter/2("Phi ")
  f(x)/1 -> Filter/1(f(x))
  Theta_hat_dot/1 -> Discontinuous_Proj_(49)/1(Theta_dot), theta dot/1
  Constant2/1 -> Switch1/2
  Gamma/1(" gamma") -> Display/1, gamma/1, Switch1/3, Divide/1
  Switch1/1 -> Theta_hat_dot/1
  Divide/1 -> Switch1/1
  Gamma/2(" 1+nu.Phi.G.Phi") -> Divide/2
  Filter/2(Phi_f) -> Epsilon/2(Phi_f), Theta_hat_dot/2, Gamma/1(Phi_f), Uf/1
  Adapt/1 -> Gamma/2(Adapt)
  Adapt1/1 -> Discontinuous_Proj_(49)/2(Adapt)

== system IARC_Nonlinear_Sensors/ARC Controller/Attitutde Control/pitch control/Adaptation Law_X/Integral Type Adaptation Law Discontinuous Projection1 ==
  Phi : Inport
  error : Inport  Port=2
  Constant : Constant  Value=gamma
  Constant2 : Constant  Value=Adaptation_ON
  Discontinuous Projection : Integrator  InitialCondition=theta0  LimitOutput=on  UpperSaturationLimit=theta_max  LowerSaturationLimit=theta_min
  InitializationDelay : UAV_Control/InitializationDelay  t0=t0
      settings: SourceProductName=UAV_Control
  Product1 : Product  Inputs=3  Multiplication=Matrix(*)
  Switch1 : Switch  Criteria=u2 ~= 0
  real : Constant  Value=theta
  theta_est : Outport
  wires:
  Constant/1 -> Product1/1
  error/1 -> Product1/3
  real/1 -> Switch1/3
  Constant2/1 -> Switch1/2
  InitializationDelay/1 -> Discontinuous Projection/1
  Product1/1 -> InitializationDelay/1
  Phi/1 -> Product1/2
  Discontinuous Projection/1 -> Switch1/1
  Switch1/1 -> theta_est/1

== system IARC_Nonlinear_Sensors/ARC Controller/Attitutde Control/pitch control/Adaptation Law_X/J ==
  Constant4 : Constant  Value=Jy
  Gain : Gain  Gain=K*L
  Math Function : Math  Operator=reciprocal  SaturateOnIntegerOverflow=on
  Step : Step  Time=I_add_time  After=I_add(2,2)  SampleTime=0
  Sum : Sum  Inputs=|++
  Out1 : Outport
  wires:
  Constant4/1 -> Sum/1
  Step/1 -> Sum/2
  Math Function/1 -> Gain/1
  Gain/1 -> Out1/1
  Sum/1 -> Math Function/1

== system IARC_Nonlinear_Sensors/ARC Controller/Attitutde Control/pitch control/Adaptation Law_X/Subsystem1 ==
  u : Inport
  6 : Scope
  Constant4 : Constant  Value=Jy
  Divide : Product  Inputs=**
  J_add : Step  Time=I_add_time  After=I_add(1,1)  SampleTime=0
  Sum : Sum  Inputs=|++
  y : Outport
  wires:
  u/1 -> Divide/1
  J_add/1 -> Sum/2
  Divide/1 -> y/1
  Sum/1 -> Divide/2, 6/1
  Constant4/1 -> Sum/1

== system IARC_Nonlinear_Sensors/ARC Controller/Attitutde Control/pitch control/Phi3/alpha 4 dot ==
  Add : Sum  Inputs=-+
  Discrete Derivative1 : simulink/Discrete/Discrete Derivative  gainval=1.0  ICPrevScaledInput=0.0  OutMin=[]  OutMax=[]  OutDataType=fixdt(1, 16)  OutScaling=2^-10  DoSatur=off
  Discrete Derivative2 : simulink/Discrete/Discrete Derivative  gainval=1.0  ICPrevScaledInput=0.0  OutMin=[]  OutMax=[]  OutDataType=fixdt(1, 16)  OutScaling=2^-10  DoSatur=off
  Sum3 : Sum  Inputs=|+-
  Transfer Fcn3 : TransferFcn  Denominator=A_2df
  k3 : Gain  Gain=k3
  alpha_4_dot : Outport
  wires:
  Discrete Derivative1/1 -> Transfer Fcn3/1
  Transfer Fcn3/1 -> Add/2
  k3/1 -> Add/1
  Discrete Derivative2/1 -> Discrete Derivative1/1
  Add/1 -> alpha_4_dot/1
  Sum3/1 -> k3/1  "ex"
  [theta] -> Sum3/1
  [theta_d] -> Discrete Derivative2/1, Sum3/2

== system IARC_Nonlinear_Sensors/ARC Controller/Attitutde Control/pitch control/f(x)/T1 .. T3 .. ==
  "  " : Trigonometry  Operator=tan
  "    " : Trigonometry
  "     " : Trigonometry  Operator=cos
  "  2" : Trigonometry  Operator=tan
  Add : Sum  Inputs=+-
  Constant : Constant  Value=Jx
  Constant1 : Constant  Value=Jyaw
  Product1 : Product  Inputs=***/
  Product2 : Product  Inputs=***/
  Out1 : Outport
  wires:
  Constant/1 -> Product1/4
  [phi] -> "  "/1
  "  "/1 -> Product1/1
  [T1] -> Product1/3
  Product2/1 -> Add/2
  [theta] -> "    "/1
  "    "/1 -> Product1/2
  Add/1 -> Out1/1
  Product1/1 -> Add/1
  "     "/1 -> Product2/2
  [theta] -> "     "/1
  "  2"/1 -> Product2/1
  [phi] -> "  2"/1
  Constant1/1 -> Product2/4
  [T3] -> Product2/3

== system IARC_Nonlinear_Sensors/ARC Controller/Attitutde Control/pitch control/f(x)/f ==
  " " : Trigonometry  Operator=sincos
  "  " : Trigonometry
  "      " : Trigonometry  Operator=tan
  Add : Sum  Inputs=+++-
  Add1 : Sum  Inputs=+-
  Constant : Constant  Value=(Jx-Jyaw)/Jy
  Constant1 : Constant  Value=(Jy-Jyaw)/Jx
  Discrete Derivative1 : simulink/Discrete/Discrete Derivative  gainval=1.0  ICPrevScaledInput=0.0  OutMin=[]  OutMax=[]  OutDataType=fixdt(1, 16)  OutScaling=2^-10  DoSatur=off
  Discrete Derivative2 : simulink/Discrete/Discrete Derivative  gainval=1.0  ICPrevScaledInput=0.0  OutMin=[]  OutMax=[]  OutDataType=fixdt(1, 16)  OutScaling=2^-10  DoSatur=off
  Discrete Derivative3 : simulink/Discrete/Discrete Derivative  gainval=1.0  ICPrevScaledInput=0.0  OutMin=[]  OutMax=[]  OutDataType=fixdt(1, 16)  OutScaling=2^-10  DoSatur=off
  Ground : Ground
  Product1 : Product
  Product2 : Product  Inputs=**/
  Product3 : Product
  Product4 : Product  Inputs=4
  Selector : Selector  InputPortWidth=3  IndexOptions=Index vector (dialog)  Indices=[1 3]  OutputSizes=1
  Selector1 : Selector  InputPortWidth=3  IndexOptions=Index vector (dialog)  Indices=[2 3]  OutputSizes=1
  p.r : Product  Inputs=*
  q.r : Product  Inputs=*
  Out1 : Outport
  wires:
  Ground/1 -> Add/3
  Product3/1 -> Add/2
  "  "/1 -> Product4/3
  [theta] -> "  "/1
  p.r/1 -> Product3/2
  Selector/1 -> p.r/1
  [pqr_est] -> Selector/1
  Constant/1 -> Product3/1
  Product2/1 -> Add/1
  Add/1 -> Out1/1
  [phi] -> Discrete Derivative1/1, " "/1
  Discrete Derivative3/1 -> Add1/1
  [psi] -> Discrete Derivative3/1
  [theta] -> Discrete Derivative2/1
  Discrete Derivative2/1 -> Product1/1
  " "/1 -> Product1/2
  Product1/1 -> Add1/2
  Add1/1 -> Product2/2
  " "/2 -> Product2/3
  Discrete Derivative1/1 -> Product2/1
  Constant1/1 -> Product4/1
  [pqr_est] -> Selector1/1
  Selector1/1 -> q.r/1
  q.r/1 -> Product4/2
  Product4/1 -> Add/4
  "      "/1 -> Product4/4
  [phi] -> "      "/1

== system IARC_Nonlinear_Sensors/ARC Controller/Attitutde Control/pitch control/phi/Notch Filter2 ==
  u : Inport
  Discrete Transfer Fcn : DiscreteTransferFcn  Numerator=an1  Denominator=bn1  SampleTime=1/500
  Discrete Transfer Fcn1 : DiscreteTransferFcn  Numerator=an2  Denominator=bn2  SampleTime=1/500
  Discrete Transfer Fcn2 : DiscreteTransferFcn  Numerator=an3  Denominator=bn3  SampleTime=1/500
  First-Order Hold : simulink/Discrete/First-Order Hold  DisableCoverage=on  Ts=1/500
      settings: SourceProductName=Simulink  SourceProductBaseCode=SL
  Mux : Mux
  Mux1 : Mux  Inputs=2
  Scope : Scope
  Scope1 : Scope
  Transfer Fcn : TransferFcn  Numerator=[60]  Denominator=[1 60]
  p : Outport
  wires:
  u/1 -> Mux1/1, Transfer Fcn/1
  Transfer Fcn/1 -> Mux1/2, First-Order Hold/1
  Discrete Transfer Fcn1/1 -> Mux/3, Discrete Transfer Fcn2/1
  First-Order Hold/1 -> Discrete Transfer Fcn/1, Mux/1
  Mux/1 -> Scope/1
  Discrete Transfer Fcn2/1 -> Mux/4, p/1
  Discrete Transfer Fcn/1 -> Mux/2, Discrete Transfer Fcn1/1
  Mux1/1 -> Scope1/1

== system IARC_Nonlinear_Sensors/ARC Controller/Attitutde Control/roll control/Adaptation Law_Y/  ==
  1 : Scope
  Constant4 : Constant  Value=Jy
  Divide : Product  Inputs=*/
  J_add : Step  Time=I_add_time  After=I_add(1,1)  SampleTime=0
  Selector : Selector  InputPortWidth=3  IndexOptions=Index vector (dialog)  Indices=1  OutputSizes=1
  Sum : Sum  Inputs=|++
  Sum1 : Sum  Inputs=++|
  T_add : Step  Time=T_add_time  After=T_add(1,1)  SampleTime=0
  Out1 : Outport
  wires:
  T_add/1 -> Sum1/2
  [Md] -> Selector/1
  Divide/1 -> 1/1, Out1/1
  Sum/1 -> Divide/2
  Constant4/1 -> Sum/1
  J_add/1 -> Sum/2
  Sum1/1 -> Divide/1
  Selector/1 -> Sum1/1

== system IARC_Nonlinear_Sensors/ARC Controller/Attitutde Control/roll control/Adaptation Law_Y/IARC, Physical Model Based Parameter Estimation (69)_roll (phi) ==
  f(x) : Inport
  Phi : Inport  Port=2
  Adapt : Inport  Port=3
  Adapt1 : InportShadow  Port=3
  Constant2 : Constant  Value=Norm_ON
  Discontinuous_Proj_(49) : Subsystem
  Display : Display  Commented=on
  Divide : Product  Inputs=*/
  Epsilon : Subsystem
  Filter : Subsystem
  Gamma : Subsystem
  Switch1 : Switch  Threshold=0.5
  Theta_hat_dot : Product  Inputs=3  Multiplication=Matrix(*)
  Uf : Scope  Commented=on
  "epsilon  " : Scope  Commented=on
  gamma : Scope  Commented=on
  theta dot : Scope  Commented=on
  theta hat : Scope  Commented=on
  Theta_hat : Outport
  wires:
  Epsilon/1(Epsilon) -> Theta_hat_dot/3, "epsilon  "/1  "predicted output error"
  Discontinuous_Proj_(49)/1(Theta) -> theta hat/1, Theta_hat/1, Epsilon/3(Theta_hat)
  Filter/1(f(x)_f) -> Epsilon/1(f(x)_f_dot)
  Phi/1 -> Filter/2("Phi ")
  f(x)/1 -> Filter/1(f(x))
  Theta_hat_dot/1 -> Discontinuous_Proj_(49)/1(Theta_dot), theta dot/1
  Constant2/1 -> Switch1/2
  Gamma/1(" gamma") -> Display/1, gamma/1, Switch1/3, Divide/1
  Switch1/1 -> Theta_hat_dot/1
  Divide/1 -> Switch1/1
  Gamma/2(" 1+nu.Phi.G.Phi") -> Divide/2
  Filter/2(Phi_f) -> Epsilon/2(Phi_f), Theta_hat_dot/2, Gamma/1(Phi_f), Uf/1
  Adapt/1 -> Gamma/2(Adapt)
  Adapt1/1 -> Discontinuous_Proj_(49)/2(Adapt)

== system IARC_Nonlinear_Sensors/ARC Controller/Attitutde Control/roll control/Adaptation Law_Y/Integral Type Adaptation Law Discontinuous Projection ==
  Phi : Inport
  error : Inport  Port=2
  Constant : Constant  Value=gamma
  Constant2 : Constant  Value=Adaptation_ON
  Discontinuous Projection : Integrator  InitialCondition=theta0  LimitOutput=on  UpperSaturationLimit=theta_max  LowerSaturationLimit=theta_min
  InitializationDelay : Subsystem  AncestorBlock=UAV_Control/InitializationDelay  mask(InitializationDelay){t0=t0}
      mask prompts: t0 "Initialization delay:"
      mask help: Applays a delay before passing the first signal.
      mask Help: Applays a delay (t0) before passing the first signal
      mask Display:
      | port_label('input',1,'u','texmode','on')
      | port_label('output',1,'y','texmode','on')
  Product1 : Product  Inputs=3  Multiplication=Matrix(*)
  Switch1 : Switch  Criteria=u2 ~= 0
  real : Constant  Value=theta
  theta_est : Outport
  wires:
  Constant/1 -> Product1/1
  error/1 -> Product1/3
  real/1 -> Switch1/3
  Constant2/1 -> Switch1/2
  InitializationDelay/1(y) -> Discontinuous Projection/1
  Product1/1 -> InitializationDelay/1(u)
  Phi/1 -> Product1/2
  Discontinuous Projection/1 -> Switch1/1
  Switch1/1 -> theta_est/1

== system IARC_Nonlinear_Sensors/ARC Controller/Attitutde Control/roll control/Adaptation Law_Y/J ==
  Constant4 : Constant  Value=Jx
  Gain : Gain  Gain=K*L
  Math Function : Math  Operator=reciprocal  SaturateOnIntegerOverflow=on
  Step : Step  Time=I_add_time  After=I_add(1,1)  SampleTime=0
  Sum : Sum  Inputs=|++
  Out1 : Outport
  wires:
  Constant4/1 -> Sum/1
  Step/1 -> Sum/2
  Math Function/1 -> Gain/1
  Gain/1 -> Out1/1
  Sum/1 -> Math Function/1

== system IARC_Nonlinear_Sensors/ARC Controller/Attitutde Control/roll control/Adaptation Law_Y/Subsystem2 ==
  u : Inport
  6 : Scope
  Constant4 : Constant  Value=Jy
  Divide : Product  Inputs=**
  J_add : Step  Time=I_add_time  After=I_add(1,1)  SampleTime=0
  Sum : Sum  Inputs=|++
  y : Outport
  wires:
  Constant4/1 -> Sum/1
  Sum/1 -> 6/1, Divide/2
  Divide/1 -> y/1
  J_add/1 -> Sum/2
  u/1 -> Divide/1

== system IARC_Nonlinear_Sensors/ARC Controller/Attitutde Control/roll control/Phi3/alpha 8 dot ==
  Add : Sum  Inputs=-+
  Discrete Derivative1 : simulink/Discrete/Discrete Derivative  gainval=1.0  ICPrevScaledInput=0.0  OutMin=[]  OutMax=[]  OutDataType=fixdt(1, 16)  OutScaling=2^-10  DoSatur=off
  Discrete Derivative2 : simulink/Discrete/Discrete Derivative  gainval=1.0  ICPrevScaledInput=0.0  OutMin=[]  OutMax=[]  OutDataType=fixdt(1, 16)  OutScaling=2^-10  DoSatur=off
  Sum3 : Sum  Inputs=|+-
  Transfer Fcn3 : TransferFcn  Denominator=A_2df
  k7 : Gain  Gain=k7
  alpha_8_dot : Outport
  wires:
  [phi_d] -> Sum3/2, Discrete Derivative2/1
  [phi] -> Sum3/1
  Sum3/1 -> k7/1  "ex"
  Add/1 -> alpha_8_dot/1
  Discrete Derivative2/1 -> Discrete Derivative1/1
  k7/1 -> Add/1
  Transfer Fcn3/1 -> Add/2
  Discrete Derivative1/1 -> Transfer Fcn3/1

== system IARC_Nonlinear_Sensors/ARC Controller/Attitutde Control/roll control/f(x)/f ==
  " " : Trigonometry  Operator=cos
  "  " : Trigonometry
  Add : Sum  Inputs=---
  Constant : Constant  Value=(Jy-Jyaw)/Jx
  Discrete Derivative2 : simulink/Discrete/Discrete Derivative  gainval=1.0  ICPrevScaledInput=0.0  OutMin=[]  OutMax=[]  OutDataType=fixdt(1, 16)  OutScaling=2^-10  DoSatur=off
  Discrete Derivative3 : simulink/Discrete/Discrete Derivative  gainval=1.0  ICPrevScaledInput=0.0  OutMin=[]  OutMax=[]  OutDataType=fixdt(1, 16)  OutScaling=2^-10  DoSatur=off
  Ground : Ground
  Product2 : Product  Inputs=3
  Product3 : Product  Inputs=3
  Selector : Selector  InputPortWidth=3  IndexOptions=Index vector (dialog)  Indices=[2 3]  OutputSizes=1
  q.r : Product  Inputs=*
  Out1 : Outport
  wires:
  [theta] -> Discrete Derivative2/1
  [psi] -> Discrete Derivative3/1
  Discrete Derivative2/1 -> Product2/1
  Discrete Derivative3/1 -> Product2/2
  [phi] -> " "/1
  " "/1 -> Product2/3
  Add/1 -> Out1/1
  Product2/1 -> Add/1
  Constant/1 -> Product3/1
  [pqr_est] -> Selector/1
  Selector/1 -> q.r/1
  q.r/1 -> Product3/2
  [theta] -> "  "/1
  "  "/1 -> Product3/3
  Product3/1 -> Add/2
  Ground/1 -> Add/3

== system IARC_Nonlinear_Sensors/ARC Controller/Attitutde Control/roll control/f(x)/s_theta.T3//Iz ==
  "  " : Trigonometry
  Constant : Constant  Value=Jyaw
  Product1 : Product  Inputs=**/
  Out1 : Outport
  wires:
  [T3] -> Product1/2
  "  "/1 -> Product1/1
  [theta] -> "  "/1
  Constant/1 -> Product1/3
  Product1/1 -> Out1/1

== system IARC_Nonlinear_Sensors/ARC Controller/Attitutde Control/roll control/phi/Notch Filter2 ==
  u : Inport
  Discrete Transfer Fcn : DiscreteTransferFcn  Numerator=an1  Denominator=bn1  SampleTime=1/500
  Discrete Transfer Fcn1 : DiscreteTransferFcn  Numerator=an2  Denominator=bn2  SampleTime=1/500
  Discrete Transfer Fcn2 : DiscreteTransferFcn  Numerator=an3  Denominator=bn3  SampleTime=1/500
  First-Order Hold : simulink/Discrete/First-Order Hold  DisableCoverage=on  Ts=1/500
      settings: SourceProductName=Simulink  SourceProductBaseCode=SL
  Mux : Mux
  Mux1 : Mux  Inputs=2
  Scope : Scope
  Scope1 : Scope
  Transfer Fcn : TransferFcn  Numerator=[60]  Denominator=[1 60]
  p : Outport
  wires:
  Mux1/1 -> Scope1/1
  Discrete Transfer Fcn/1 -> Discrete Transfer Fcn1/1, Mux/2
  Discrete Transfer Fcn2/1 -> p/1, Mux/4
  Mux/1 -> Scope/1
  First-Order Hold/1 -> Mux/1, Discrete Transfer Fcn/1
  Discrete Transfer Fcn1/1 -> Discrete Transfer Fcn2/1, Mux/3
  Transfer Fcn/1 -> First-Order Hold/1, Mux1/2
  u/1 -> Transfer Fcn/1, Mux1/1
